simulink model "ssSim"  (R2024a)
settings: Solver=VariableStepAuto  StartTime=0.0  StopTime=10.0  RelTol=1e-3
values from neighbouring files (symbols this model uses):
  A = [ ... (first row only)    [main.m]
  B = [0; 0; 1]    [main.m]
  C = [1 0 0 ]    [main.m]
  I = [ 1 0 0; 0 1 0; 0 0 1]    [main.m]
  Kd = 1/dcgain(Gc)    [main.m]
  ks = [kb(1), kb(2), kb(3)]    [main.m]
settings Model: Creator=jvsb2  LastModifiedBy=jvsb2

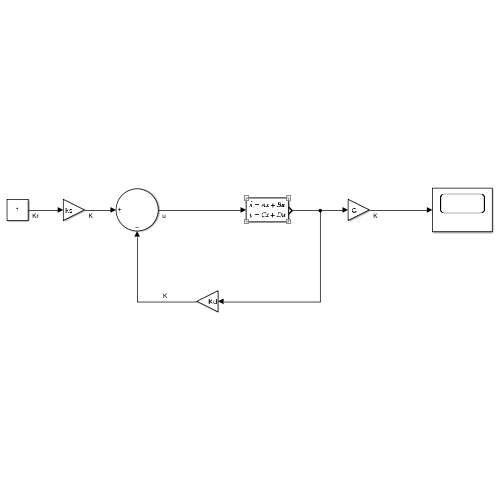
[thumbnail: Simulink's stored preview of the top-level diagram]
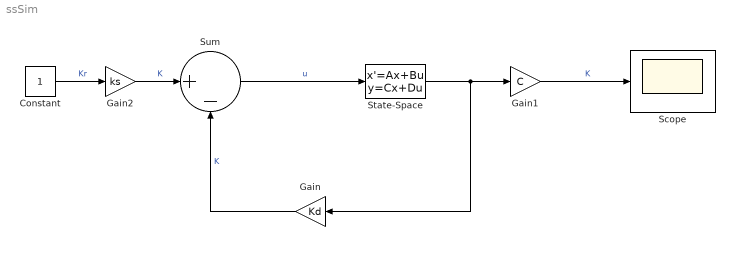
== system ssSim ==
  Constant : Constant
  Gain : Gain  Gain=Kd
  Gain1 : Gain  Gain=C
  Gain2 : Gain  Gain=ks
  Scope : Scope
  State-Space : StateSpace  A=A  B=B  C=I  D=[0; 0; 0]  InitialCondition=0
  Sum : Sum  Inputs=|+-
  wires:
  Gain/1 -> Sum/2  "K"
  Sum/1 -> State-Space/1  "u"
  Constant/1 -> Gain2/1  "Kr"
  Gain2/1 -> Sum/1  "K"
  State-Space/1 -> Gain/1, Gain1/1
  Gain1/1 -> Scope/1  "K"
